simulink model "serial_paralel_feedback"  (R2019a)
settings: Solver=VariableStepAuto  StartTime=0.0  StopTime=10.0  RelTol=1e-3
model workspace (MAT data in the model file):
  A_1 = 1
  A_2 = 1
  B_1 = 1
  B_2 = 1
settings Model: Creator=ASROCK  LastModifiedBy=Martin Dodek
settings DataIOCC: ReturnWorkspaceOutputs=off
settings DebuggingCC: ArithmeticOperatorsInVariantConditions=warning
settings SFSimCC: SimUseLocalCustomCode=off
settings RTWCC: RTWUseLocalCustomCode=off

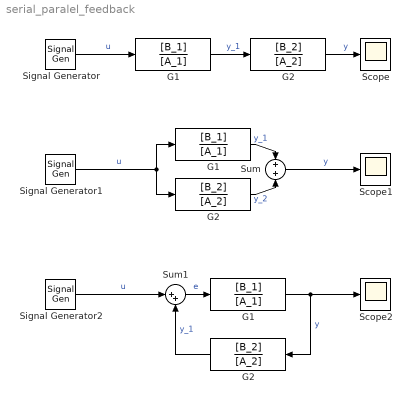
== system serial_paralel_feedback ==
  G1 : TransferFcn  Numerator=[B_1]  Denominator=[A_1]
  "G1 " : TransferFcn  Numerator=[B_1]  Denominator=[A_1]
  "G1 " : TransferFcn  Numerator=[B_1]  Denominator=[A_1]
  G2 : TransferFcn  Numerator=[B_2]  Denominator=[A_2]
  "G2 " : TransferFcn  Numerator=[B_2]  Denominator=[A_2]
  "G2 " : TransferFcn  Numerator=[B_2]  Denominator=[A_2]
  Scope : Scope
  Scope1 : Scope
  Scope2 : Scope
  Signal Generator : SignalGenerator  Units=rad/sec
  Signal Generator1 : SignalGenerator  Units=rad/sec
  Signal Generator2 : SignalGenerator  Units=rad/sec
  Sum : Sum
  Sum1 : Sum  Inputs=|++
  wires:
  G1/1 -> G2/1  "y_1"
  Signal Generator/1 -> G1/1  "u"
  G2/1 -> Scope/1  "y"
  "G2 "/1 -> Sum/2  "y_2"
  "G1 "/1 -> Sum/1  "y_1"
  Signal Generator1/1 -> "G2 "/1, "G1 "/1  "u"
  Sum/1 -> Scope1/1  "y"
  Sum1/1 -> "G1 "/1  "e"
  Signal Generator2/1 -> Sum1/1  "u"
  "G2 "/1 -> Sum1/2  "y_1"
  "G1 "/1 -> Scope2/1, "G2 "/1  "y"
